simulink model "generacion"  (R2025a)
settings: Solver=VariableStepAuto  StartTime=0.0  StopTime=10.0  RelTol=1e-3
settings Model: Creator=arnavk  LastModifiedBy=arnavk

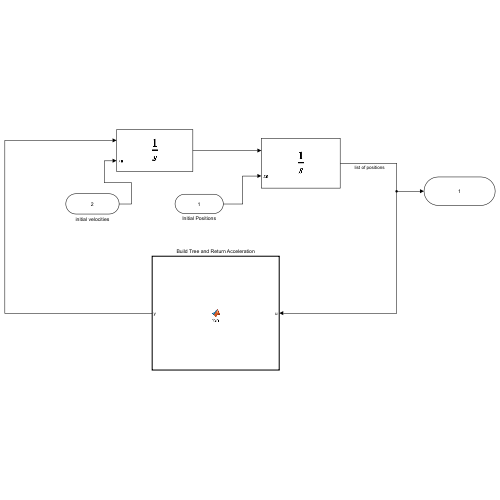
[thumbnail: Simulink's stored preview of the top-level diagram]
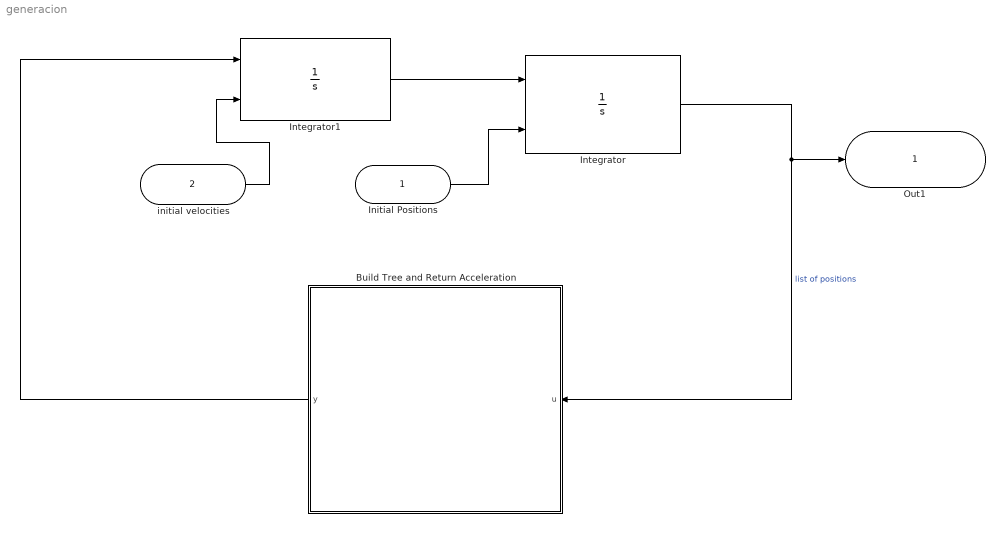
== system generacion ==
  Initial Positions : Inport
  initial velocities : Inport  Port=2
  Build Tree and Return Acceleration : MATLAB Function  TreatAsAtomicUnit=on
  Integrator : Integrator  InitialConditionSource=external
  Integrator1 : Integrator  InitialConditionSource=external
  Out1 : Outport
  wires:
  Integrator/1 -> Build Tree and Return Acceleration/1(u), Out1/1  "list of positions"
  Integrator1/1 -> Integrator/1
  Build Tree and Return Acceleration/1(y) -> Integrator1/1
  Initial Positions/1 -> Integrator/2
  initial velocities/1 -> Integrator1/2

== matlab function generacion/Build Tree and Return Acceleration ==
  data: u input; y output
function y = fcn(u)

y = u;
